simulink model "DC-DC Boost Converter Simscape SIMULINK"  (R2022b)
settings: Solver=VariableStepAuto  StartTime=0.0  StopTime=0.1  RelTol=1e-3
values from neighbouring files (symbols this model uses):
  C = 1e-3    (= 0.001)    [Boost_Converter_Parameters.m]
  Dnom = 0.55    [Boost_Converter_Parameters.m]
  fS = 10^5    (= 100000)    [Boost_Converter_Parameters.m]
  L = 100e-6    (= 0.0001)    [Boost_Converter_Parameters.m]
  rC = 0.01    [Boost_Converter_Parameters.m]
  rL = 0.08    [Boost_Converter_Parameters.m]
  RL = 4.5    [Boost_Converter_Parameters.m]
  Vinnom = 24    [Boost_Converter_Parameters.m]
libraries: spsSeriesRLCBranchLib x3, spsControlledVoltageSourceLib x1, spsCurrentMeasurementLib x1, spsDiodeLib x1, spsMosfetLib x1, spsVoltageMeasurementLib x1, sps_lib x1
settings Model: Creator=YESHIWAS  LastModifiedBy=YESHIWAS
settings DataIOCC: ReturnWorkspaceOutputs=off

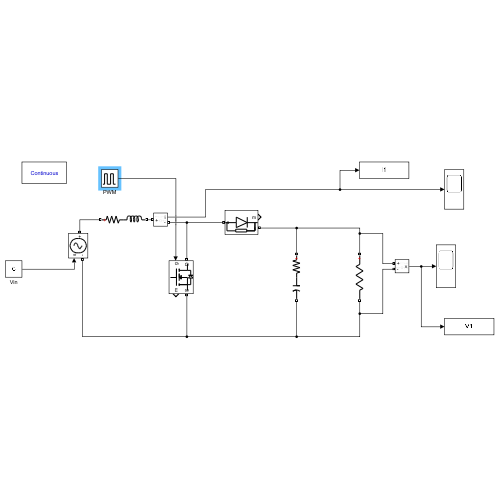
[thumbnail: Simulink's stored preview of the top-level diagram]
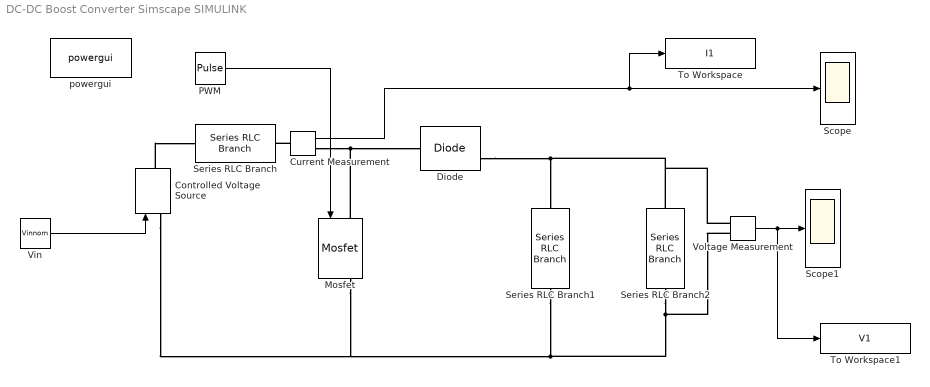
== system DC-DC Boost Converter Simscape SIMULINK ==
  Controlled Voltage Source : spsControlledVoltageSourceLib/Controlled Voltage Source  Initialize=on  Source_Type=AC  Amplitude=0  Phase=0  Frequency=0  Measurements=None
  Current Measurement : spsCurrentMeasurementLib/Current Measurement  PhasorSimulation=off  OutputType=Complex  PSBequivalent=0
  Diode : spsDiodeLib/Diode  Ron=RF  Lon=0  Vf=VF  IC=0  UseSnubber=0  Rs=500  Cs=250e-9  Measurements=on
  Mosfet : spsMosfetLib/Mosfet  Ron=rDS  Lon=0  Rd=0.01  Vfd=0  IC=0  Rs=1e5  Cs=inf  Measurements=on
  PWM : DiscretePulseGenerator  PulseType=Time based  Period=1/fS  PulseWidth=Dnom*100
  Scope : Scope
  Scope1 : Scope
  Series RLC Branch : spsSeriesRLCBranchLib/Series RLC Branch  LConnTagsString=__new0  RConnTagsString=__new0  BranchType=RL  Resistance=rL  Inductance=L  SetiL0=off  InitialCurrent=0  Capacitance=1e-6  Setx0=off  InitialVoltage=0  Measurements=None
  Series RLC Branch1 : spsSeriesRLCBranchLib/Series RLC Branch  LConnTagsString=__new0  RConnTagsString=__new0  BranchType=RC  Resistance=rC  Inductance=1e-3  SetiL0=off  InitialCurrent=0  Capacitance=C  Setx0=off  InitialVoltage=0  Measurements=None
  Series RLC Branch2 : spsSeriesRLCBranchLib/Series RLC Branch  LConnTagsString=__new0  RConnTagsString=__new0  BranchType=R  Resistance=RL  Inductance=1e-3  SetiL0=off  InitialCurrent=0  Capacitance=1e-6  Setx0=off  InitialVoltage=0  Measurements=None
  To Workspace : ToWorkspace  VariableName=I1  SaveFormat=Structure With Time  SampleTime=-1
  To Workspace1 : ToWorkspace  VariableName=V1  SaveFormat=Structure With Time  SampleTime=-1
  Vin : Constant  Value=Vinnom  SampleTime=0.001
  Voltage Measurement : spsVoltageMeasurementLib/Voltage Measurement  PhasorSimulation=off  OutputType=Complex  PSBequivalent=0
  powergui : sps_lib/powergui  Priority=1  SimulationMode=Continuous  SampleTime=50e-6  frequency=60  Iterations=50  frequencyindice=0  Pbase=100e6  ErrMax=1e-4  UnitsV=kV  UnitsW=MW  buscounter=0  FunctionMessages=off  echomessages=off  EnableUseOfTLC=off  CurrentSourceSwitches=off  DisableSnubberDevices=off  DisableRonSwitches=off  DisableVfSwitches=off  DisplayEquations=off  AutomaticDiscreteSolvers=off  SolverType=Tustin/Backward Euler (TBE)  Interpol=off  ExternalGateDelay=off  methode=off  Ts=100  x0status=blocks  SPID=on  SwTol=0  HookPort=off  NonlinearTolerance=1e-4  nMaxIteration=100  ContinueOnMaxIteration=off  RestoreLinks=warning  ResistiveCurrentMeasurement=off  Frange=[0:2:500]  Ylog=off  Xlog=on  ShowGrid=off  save=off  variable=ZData  structure=0  ZoomFFT=off  StartTime=0.0  cycles=1  DisplayStyle=1  fundamental=60  FreqAxis=off  MaxFrequency=1000  frequencyindicesteady=1  RmsSteady=1  display=off
  wires:
  Vin/1 -> Controlled Voltage Source/1
  Voltage Measurement/1 -> To Workspace1/1, Scope1/1
  Current Measurement/1 -> To Workspace/1, Scope/1
  PWM/1 -> Mosfet/1
  connections:
  Series RLC Branch2/RConn1 -- Voltage Measurement/LConn2 -- Mosfet/RConn1 -- Controlled Voltage Source/LConn1 -- Series RLC Branch1/RConn1
  Voltage Measurement/LConn1 -- Series RLC Branch2/LConn1 -- Diode/RConn1 -- Series RLC Branch1/LConn1
  Controlled Voltage Source/RConn1 -- Series RLC Branch/LConn1
  Mosfet/LConn1 -- Current Measurement/RConn1 -- Diode/LConn1
  Current Measurement/LConn1 -- Series RLC Branch/RConn1
